simulink model "EV_Pwr_Manager"  (R2013b)
settings: Solver=FixedStepDiscrete  StartTime=0.0  StopTime=inf  RelTol=1e-3
InitFcn:
  | %EV_Param_Update
  | % update the number of strings (discretized)
  | numStrings = round(Opti_numStrings);
  | %disp(['Number of strings: ' num2str(numStrings)])
  | % update the effective capacity based on the number of strings
  | EV_Param.Battery_Det.Rated_Capacity = 28.5*numStrings; %A*hr
  | EV_Param.Battery_Det.DP = 1.5*fliplr([1500 1500 1600 1450 1325 1125 925 675 425 175 ])./8*EV_Param.Battery_Det.Rated_Capacity; % 8 comes from the 8Ahr rated batter data used (normalize and rescale to the rated capacity
  | EV_Param.Battery_Det.CP = fliplr([25 100 200 250 375 550 750 950 1125 1150])./8*EV_Param.Battery_Det.Rated_Capacity;
  | 
  | % update the number of cells in a string (discretized)
  | numSeriesCells = round(Opti_numSeriesCells);
  | %disp(['Number of cells in a string: ' num2str(numSeriesCells)])
  | % update the nominal string volage and charge deficit
  | EV_Param.Battery_Det.Nominal_Voltage = numSeriesCells*cellVolts;
  | BatteryParams(1).Qe_init = 0;%EV_Param.Battery_Det.Rated_Capacity*(1-EV_Param.Battery_Det.Initial_SOC/100); %Ampere*hours
  | 
  | % update the total number of cells, battery pack mass and total vehicle
  | % mass
  | total_cells = numSeriesCells*numStrings;
  | %disp(['Total Number of cells: ' num2str(total_cells)])
  | EV_Param.BatteryMass = BatteryParams(1).cell_mass*total_cells;
  | %disp(['Total Battery Pack Mass: ' num2str(EV_Param.BatteryMass)])
  | EV_Param.Vehicle.Mass = 1300+EV_Param.BatteryMass;
  | 
  | % update the driveline gear ratio
  | EV_Param.Vehicle.Engine_Vehicle_Gear_Ratio = Opti_Vehicle_Gear_Ratio;
  | %disp(['Driveline gear ratio: ' num2str(Opti_Vehicle_Gear_Ratio)])
  | %disp('EV_Pwr_Manager has been initialized')
values from neighbouring files (symbols this model uses):
  ctrlConst = struct    [applicationData.m]
undefined symbols (not defined in the file or in its folder): brake_cmd_table, decel_cmd_vec, DiscIntNeverNeededParam, Motor_Limits, Motor_Spd_Ref_radps, regen_pwr_vec
libraries: simulink x13
settings Model: PauseTimes=13.1  Creator=rchladny  LastModifiedBy=rchladny
settings DataIOCC: SaveOutput=off  SaveTime=off
settings OptimizationCC: InlineParams=on  UseSpecifiedMinMax=on  ZeroExternalMemoryAtStartup=off  NoFixptDivByZeroProtection=on  EfficientFloat2IntCast=on  OptimizeModelRefInitCode=on  LifeSpan=Inf
settings DebuggingCC: InheritedTsInSrcMsg=none  ParameterPrecisionLossMsg=none  UnknownTsInhSupMsg=none
settings HardwareCC: ProdBitPerChar=16  ProdBitPerInt=16  ProdBitPerPointer=16  ProdLargestAtomicInteger=Integer  ProdIntDivRoundTo=Zero  ProdEndianess=LittleEndian  ProdWordSize=16  ProdHWDeviceType=Texas Instruments->C2000  TargetLongLongMode=on  TargetIntDivRoundTo=Zero  TargetEndianess=LittleEndian  TargetHWDeviceType=Generic->MATLAB Host Computer  ProdEqTarget=off
settings ModelReferenceCC: ModelReferenceNumInstancesAllowed=Single
settings RTWCC: SystemTargetFile=ert.tlc  TemplateMakefile=ert_default_tmf  Description=Embedded Coder  ProcessScript=ert_make_rtw_hook
settings CodeAppCC: IgnoreCustomStorageClasses=off
settings ERTTargetCC: CodeReplacementLibrary=ANSI_C  GenerateSampleERTMain=on  ERTCustomFileTemplate=example_file_process.tlc

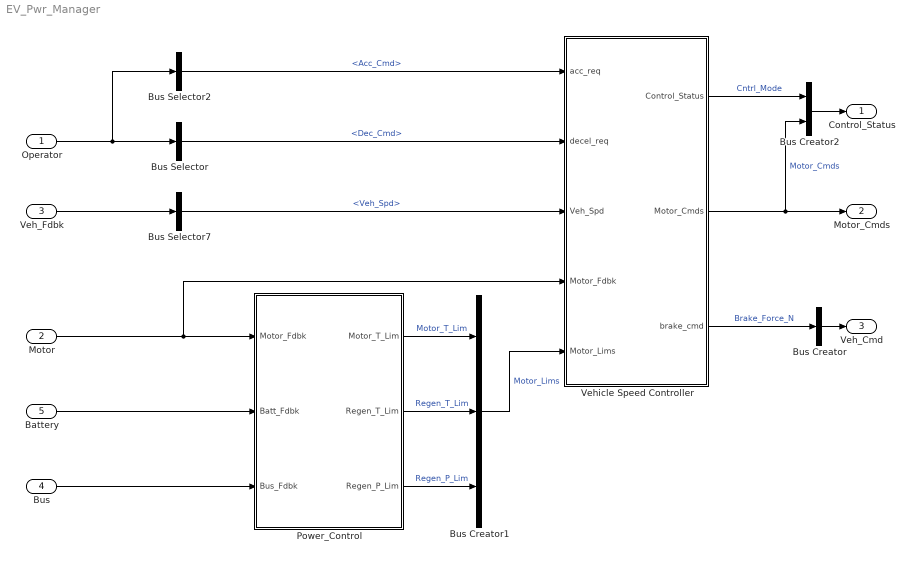
== system EV_Pwr_Manager ==
  Operator : Inport  OutDataTypeStr=Bus: Op_Cmds
  Motor : Inport  Port=2  OutDataTypeStr=Bus: Motor_Sys_Fdbk  BusOutputAsStruct=on
  Veh_Fdbk : Inport  Port=3  OutDataTypeStr=Bus: Veh_Fdbk
  Bus : Inport  Port=4  OutDataTypeStr=Bus: Bus_Fdbk  BusOutputAsStruct=on
  Battery : Inport  Port=5  OutDataTypeStr=Bus: Batt_Fdbk  BusOutputAsStruct=on
  Bus Creator : BusCreator  Inputs=1
  Bus Creator1 : BusCreator  Inputs=3
  Bus Creator2 : BusCreator  Inputs=2
  Bus Selector : BusSelector  OutputSignals=Dec_Cmd
  Bus Selector2 : BusSelector  OutputSignals=Acc_Cmd
  Bus Selector7 : BusSelector  OutputSignals=Veh_Spd
  Power_Control : Subsystem
  Vehicle Speed Controller : Subsystem
  Control_Status : Outport  OutDataTypeStr=Bus: Cntrl_Status
  Motor_Cmds : Outport  Port=2  OutDataTypeStr=Bus: Motor_Cmds
  Veh_Cmd : Outport  Port=3  OutDataTypeStr=Bus: Veh_Cmds
  wires:
  Vehicle Speed Controller/2(Motor_Cmds) -> Bus Creator2/2, Motor_Cmds/1  "Motor_Cmds"
  Power_Control/1(Motor_T_Lim) -> Bus Creator1/1  "Motor_T_Lim"
  Power_Control/2(Regen_T_Lim) -> Bus Creator1/2  "Regen_T_Lim"
  Bus Creator1/1 -> Vehicle Speed Controller/5(Motor_Lims)  "Motor_Lims"
  Power_Control/3(Regen_P_Lim) -> Bus Creator1/3  "Regen_P_Lim"
  Motor/1 -> Vehicle Speed Controller/4(Motor_Fdbk), Power_Control/1(Motor_Fdbk)
  Battery/1 -> Power_Control/2(Batt_Fdbk)
  Bus/1 -> Power_Control/3(Bus_Fdbk)
  Vehicle Speed Controller/1(Control_Status) -> Bus Creator2/1  "Cntrl_Mode"
  Veh_Fdbk/1 -> Bus Selector7/1
  Bus Creator2/1 -> Control_Status/1
  Bus Selector/1 -> Vehicle Speed Controller/2(decel_req)  "<Dec_Cmd>"
  Bus Selector2/1 -> Vehicle Speed Controller/1(acc_req)  "<Acc_Cmd>"
  Operator/1 -> Bus Selector2/1, Bus Selector/1
  Vehicle Speed Controller/3(brake_cmd) -> Bus Creator/1  "Brake_Force_N"
  Bus Creator/1 -> Veh_Cmd/1
  Bus Selector7/1 -> Vehicle Speed Controller/3(Veh_Spd)  "<Veh_Spd>"

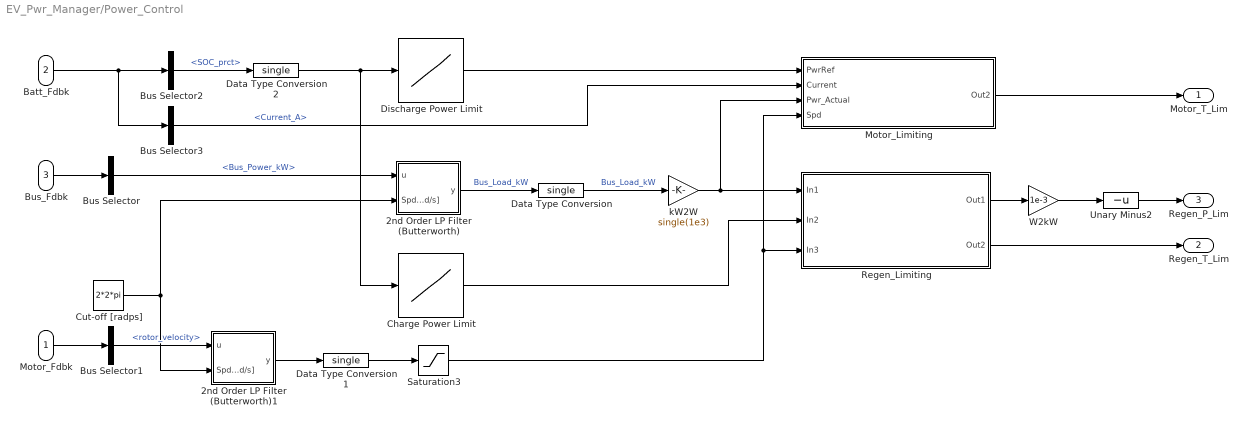
== system EV_Pwr_Manager/Power_Control ==
  Motor_Fdbk : Inport  OutDataTypeStr=Bus: Motor_Sys_Fdbk
  Batt_Fdbk : Inport  Port=2  OutDataTypeStr=Bus: Batt_Fdbk
  Bus_Fdbk : Inport  Port=3  OutDataTypeStr=Bus: Bus_Fdbk
  2nd Order LP Filter (Butterworth) : Subsystem  mask{DT=EV_Param.Control.Pwr_Cntrl_TS}
      mask prompts: DT "Sampe Time"
      mask Display:
      | plot([0 0],[0 1]);
      | plot([0 1],[0 0]);
      | plot([0 .5 .75 1],[1 1 .7071 .01]);
  2nd Order LP Filter (Butterworth)1 : Subsystem  mask{DT=EV_Param.Control.Pwr_Cntrl_TS}
      mask prompts: DT "Sampe Time"
      mask Display:
      | plot([0 0],[0 1]);
      | plot([0 1],[0 0]);
      | plot([0 .5 .75 1],[1 1 .7071 .01]);
  Bus Selector : BusSelector  OutputSignals=Bus_Power_kW
  Bus Selector1 : BusSelector  OutputSignals=Motor_Fdbk.rotor_velocity
  Bus Selector2 : BusSelector  OutputSignals=SOC_prct
  Bus Selector3 : BusSelector  OutputSignals=Current_A
  Charge Power Limit : Lookup_n-D  NumberOfTableDimensions=1  BreakpointsForDimension1=EV_Param.Battery_Det.SOC  BeginIndexSearchUsingPreviousIndexResult=on  Table=EV_Param.Battery_Det.CP  InternalRulePriority=Speed  RndMeth=Simplest  InputSameDT=on
  Cut-off [radps] : Constant  Value=2*2*pi  OutDataTypeStr=single  SampleTime=-1
  Data Type Conversion : DataTypeConversion  OutDataTypeStr=single
  Data Type Conversion1 : DataTypeConversion  OutDataTypeStr=single
  Data Type Conversion2 : DataTypeConversion  OutDataTypeStr=single
  Discharge Power Limit : Lookup_n-D  NumberOfTableDimensions=1  BreakpointsForDimension1=EV_Param.Battery_Det.SOC  BeginIndexSearchUsingPreviousIndexResult=on  Table=EV_Param.Battery_Det.DP  ExtrapMethod=Clip  UseLastTableValue=on  InternalRulePriority=Speed  RndMeth=Simplest  InputSameDT=on
  Motor_Limiting : Subsystem
  Regen_Limiting : Subsystem
  Saturation3 : Saturate  UpperLimit=inf  LowerLimit=100*pi/30
  Unary Minus2 : UnaryMinus
  W2kW : Gain  Gain=1e-3
  kW2W : Gain  Gain=single(1e3)
  Motor_T_Lim : Outport
  Regen_T_Lim : Outport  Port=2
  Regen_P_Lim : Outport  Port=3
  wires:
  Batt_Fdbk/1 -> Bus Selector3/1, Bus Selector2/1
  Cut-off [radps]/1 -> 2nd Order LP Filter (Butterworth)1/2(Spd_Err_Filt_BW [rad/s]), 2nd Order LP Filter (Butterworth)/2(Spd_Err_Filt_BW [rad/s])
  kW2W/1 -> Motor_Limiting/3(Pwr_Actual), Regen_Limiting/1(In1)
  W2kW/1 -> Unary Minus2/1
  Unary Minus2/1 -> Regen_P_Lim/1
  Saturation3/1 -> Motor_Limiting/4(Spd), Regen_Limiting/3(In3)
  Bus_Fdbk/1 -> Bus Selector/1
  2nd Order LP Filter (Butterworth)/1(y) -> Data Type Conversion/1  "Bus_Load_kW"
  Data Type Conversion/1 -> kW2W/1  "Bus_Load_kW"
  Bus Selector/1 -> 2nd Order LP Filter (Butterworth)/1(u)  "<Bus_Power_kW>"
  Motor_Fdbk/1 -> Bus Selector1/1
  Bus Selector1/1 -> 2nd Order LP Filter (Butterworth)1/1(u)  "<rotor_velocity>"
  Bus Selector2/1 -> Data Type Conversion2/1  "<SOC_prct>"
  2nd Order LP Filter (Butterworth)1/1(y) -> Data Type Conversion1/1
  Data Type Conversion1/1 -> Saturation3/1
  Data Type Conversion2/1 -> Charge Power Limit/1, Discharge Power Limit/1
  Discharge Power Limit/1 -> Motor_Limiting/1(PwrRef)
  Bus Selector3/1 -> Motor_Limiting/2(Current)  "<Current_A>"
  Motor_Limiting/1(Out2) -> Motor_T_Lim/1
  Charge Power Limit/1 -> Regen_Limiting/2(In2)
  Regen_Limiting/1(Out1) -> W2kW/1
  Regen_Limiting/2(Out2) -> Regen_T_Lim/1

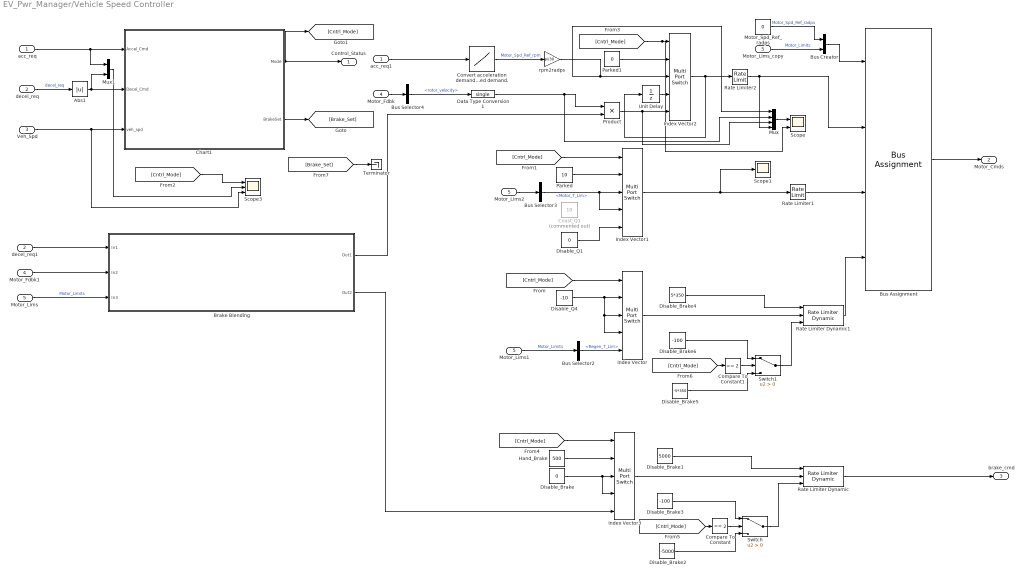
== system EV_Pwr_Manager/Vehicle Speed Controller ==
  acc_req : Inport
  decel_req : Inport  Port=2
  Veh_Spd : Inport  Port=3  OutDataTypeStr=single
  Motor_Fdbk : Inport  Port=4
  Motor_Lims : Inport  Port=5
  Abs1 : Abs
  Brake Blending : Subsystem
  Bus Assignment : BusAssignment  AssignedSignals=Motor_Spd_Ref_radps,Motor_Limits.Motor_T_Lim,Motor_Limits.Regen_T_Lim
  Bus Creator : BusCreator  Inputs=2
  Bus Selector2 : BusSelector  OutputSignals=Regen_T_Lim
  Bus Selector3 : BusSelector  OutputSignals=Motor_T_Lim
  Bus Selector4 : BusSelector  OutputSignals=Motor_Fdbk.rotor_velocity
  Chart1 : Stateflow chart  TreatAsAtomicUnit=on
  Coast_Q1 : Constant  Commented=on  Value=10  OutDataTypeStr=single
  Compare To Constant : simulink/Logic and Bit Operations/Compare To Constant  relop===  const=2  OutDataTypeStr=boolean
  Compare To Constant1 : simulink/Logic and Bit Operations/Compare To Constant  relop===  const=2  OutDataTypeStr=boolean
  Convert acceleration demand to motor speed demand. : Lookup_n-D  NumberOfTableDimensions=1  BreakpointsForDimension1=[0 1]  BeginIndexSearchUsingPreviousIndexResult=on  Table=[0 2500]*.8  InputSameDT=on
  Data Type Conversion1 : DataTypeConversion  OutDataTypeStr=single
  Disable_Brake : Constant  Value=0  OutDataTypeStr=single
  Disable_Brake1 : Constant  Value=5000  OutDataTypeStr=single  SampleTime=-1
  Disable_Brake2 : Constant  Value=-5000  OutDataTypeStr=single  SampleTime=-1
  Disable_Brake3 : Constant  Value=-100  OutDataTypeStr=single  SampleTime=-1
  Disable_Brake4 : Constant  Value=5*350  OutDataTypeStr=single  SampleTime=-1
  Disable_Brake5 : Constant  Value=-5*350  OutDataTypeStr=single  SampleTime=-1
  Disable_Brake6 : Constant  Value=-100  OutDataTypeStr=single  SampleTime=-1
  Disable_Q1 : Constant  Value=0  OutDataTypeStr=single
  Disable_Q4 : Constant  Value=-10  OutDataTypeStr=single
  Hand_Brake : Constant  Value=500  OutDataTypeStr=single
  Index Vector{,1..3} (4 alike) : MultiPortSwitch  DataPortOrder=Zero-based contiguous  Inputs=4  zeroidx=on
  Motor_Fdbk1 : InportShadow  Port=4
  Motor_Lims1 : InportShadow  Port=5
  Motor_Lims2 : InportShadow  Port=5
  Motor_Lims_copy : InportShadow  Port=5
  Motor_Spd_Ref_radps : Constant  Value=0  OutDataTypeStr=single
  Mux : Mux
  Mux1 : Mux  Inputs=2
  Parked : Constant  Value=10  OutDataTypeStr=single
  Parked1 : Constant  Value=0  OutDataTypeStr=single
  Product : Product
  Rate Limiter Dynamic : simulink/Discontinuities/Rate Limiter Dynamic
  Rate Limiter Dynamic1 : simulink/Discontinuities/Rate Limiter Dynamic
  Rate Limiter1 : RateLimiter  RisingSlewLimit=350*5  FallingSlewLimit=-350*5  SampleTimeMode=inherited
  Rate Limiter2 : RateLimiter  RisingSlewLimit=2000  FallingSlewLimit=-70  SampleTimeMode=inherited
  Scope : Scope  NumInputPorts=2
      settings: YMin=-50~-5  YMax=900~5
  Scope1 : Scope
  Scope3 : Scope  NumInputPorts=3
      settings: YMin=0~0~0  YMax=1~1~275  SaveName=ScopeData23
  Switch : Switch  Criteria=u2 > Threshold
  Switch1 : Switch  Criteria=u2 > Threshold
  Terminator : Terminator
  Unit Delay : UnitDelay  SampleTime=-1
  acc_req1 : InportShadow
  decel_req1 : InportShadow  Port=2
  rpm2radps : Gain  Gain=pi/30
  Control_Status : Outport  InitialOutput=0
  Motor_Cmds : Outport  Port=2  OutDataTypeStr=Bus: Motor_Cmds
  brake_cmd : Outport  Port=3  InitialOutput=0
  wires:
  rpm2radps/1 -> Index Vector2/3, Mux/1
  decel_req/1 -> Abs1/1  "decel_req"
  Convert acceleration demand to motor speed demand./1 -> rpm2radps/1  "Motor_Spd_Ref_rpm"
  Chart1/1(Mode) -> [Cntrl_Mode], Control_Status/1
  Chart1/2(BrakeSet) -> [Brake_Set]
  acc_req/1 -> Mux1/1, Chart1/1(Accel_Cmd)
  Abs1/1 -> Mux1/2, Chart1/2(Decel_Cmd)
  Veh_Spd/1 -> Scope3/3, Chart1/3(veh_spd)
  Motor_Lims_copy/1 -> Bus Creator/2  "Motor_Limits"
  Bus Assignment/1 -> Motor_Cmds/1
  Motor_Spd_Ref_radps/1 -> Bus Creator/1  "Motor_Spd_Ref_radps"
  Bus Creator/1 -> Bus Assignment/1
  Index Vector/1 -> Rate Limiter Dynamic1/2
  Disable_Q4/1 -> Index Vector/4, Index Vector/3, Index Vector/2
  [Cntrl_Mode] -> Index Vector/1
  Rate Limiter Dynamic1/1 -> Bus Assignment/4
  [Cntrl_Mode] -> Index Vector1/1
  Index Vector1/1 -> Scope1/1, Rate Limiter1/1
  Rate Limiter1/1 -> Bus Assignment/3
  Parked/1 -> Index Vector1/2
  [Cntrl_Mode] -> Scope/2, Index Vector2/1
  Parked1/1 -> Index Vector2/2
  Index Vector2/1 -> Unit Delay/1, Rate Limiter2/1
  Bus Selector4/1 -> Data Type Conversion1/1  "<rotor_velocity>"
  Motor_Lims1/1 -> Bus Selector2/1  "Motor_Limits"
  Bus Selector2/1 -> Index Vector/5  "<Regen_T_Lim>"
  Motor_Lims2/1 -> Bus Selector3/1
  Bus Selector3/1 -> Index Vector1/4, Index Vector1/3  "<Motor_T_Lim>"
  Product/1 -> Mux/3, Index Vector2/5
  Mux1/1 -> Scope3/2
  Index Vector3/1 -> Rate Limiter Dynamic/2
  Disable_Brake/1 -> Index Vector3/3, Index Vector3/4
  [Cntrl_Mode] -> Index Vector3/1
  Hand_Brake/1 -> Index Vector3/2
  Rate Limiter2/1 -> Mux/4, Bus Assignment/2
  [Cntrl_Mode] -> Scope3/1
  Motor_Fdbk/1 -> Bus Selector4/1
  Data Type Conversion1/1 -> Product/1, Mux/2
  Rate Limiter Dynamic/1 -> brake_cmd/1
  Switch/1 -> Rate Limiter Dynamic/3
  Compare To Constant/1 -> Switch/2
  [Cntrl_Mode] -> Compare To Constant/1
  Disable_Brake1/1 -> Rate Limiter Dynamic/1
  Disable_Brake2/1 -> Switch/3
  Disable_Brake3/1 -> Switch/1
  Switch1/1 -> Rate Limiter Dynamic1/3
  Compare To Constant1/1 -> Switch1/2
  [Cntrl_Mode] -> Compare To Constant1/1
  Disable_Brake4/1 -> Rate Limiter Dynamic1/1
  Disable_Brake5/1 -> Switch1/3
  Disable_Brake6/1 -> Switch1/1
  Disable_Q1/1 -> Index Vector1/5
  decel_req1/1 -> Brake Blending/1(In1)
  Motor_Fdbk1/1 -> Brake Blending/2(In2)
  Motor_Lims/1 -> Brake Blending/3(In3)  "Motor_Limits"
  Brake Blending/1(Out1) -> Product/2
  Brake Blending/2(Out2) -> Index Vector3/5
  [Brake_Set] -> Terminator/1
  Mux/1 -> Scope/1
  Unit Delay/1 -> Index Vector2/4
  acc_req1/1 -> Convert acceleration demand to motor speed demand./1

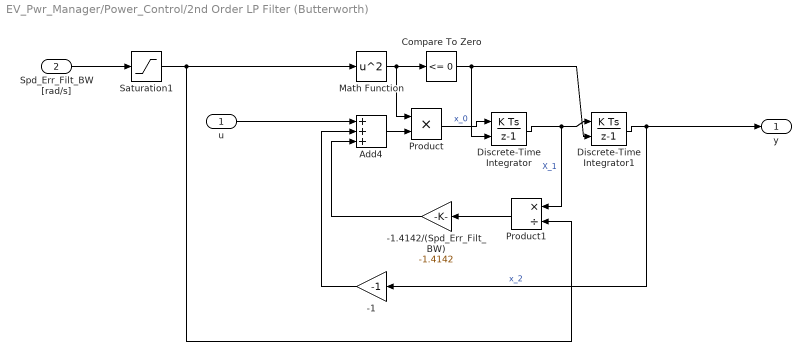
== system EV_Pwr_Manager/Power_Control/2nd Order LP Filter (Butterworth) ==
  u : Inport
  Spd_Err_Filt_BW [rad/s] : Inport  Port=2
  -1 : Gain  Gain=-1
  -1.4142/(Spd_Err_Filt_BW) : Gain  Gain=-1.4142
  Add4 : Sum  Inputs=+++
  Compare To Zero : simulink/Logic and Bit Operations/Compare To Zero  relop=<=  OutDataTypeStr=uint8
  Discrete-Time Integrator : DiscreteIntegrator  ExternalReset=rising  SampleTime=DT  ICPrevOutput=DiscIntNeverNeededParam  ICPrevScaledInput=DiscIntNeverNeededParam
  Discrete-Time Integrator1 : DiscreteIntegrator  ExternalReset=rising  SampleTime=DT  ICPrevOutput=DiscIntNeverNeededParam  ICPrevScaledInput=DiscIntNeverNeededParam
  Math Function : Math  Operator=square  SaturateOnIntegerOverflow=on
  Product : Product  RndMeth=Zero
  Product1 : Product  Inputs=*/  RndMeth=Zero
  Saturation1 : Saturate  UpperLimit=2*pi*5000  LowerLimit=.001
  y : Outport
  wires:
  Add4/1 -> Product/2
  Discrete-Time Integrator/1 -> Product1/1, Discrete-Time Integrator1/1  "X_1"
  Discrete-Time Integrator1/1 -> -1/1, y/1  "x_2"
  -1.4142/(Spd_Err_Filt_BW)/1 -> Add4/3
  -1/1 -> Add4/2
  Product/1 -> Discrete-Time Integrator/1  "x_0"
  u/1 -> Add4/1
  Math Function/1 -> Product/1, Compare To Zero/1
  Spd_Err_Filt_BW [rad/s]/1 -> Saturation1/1
  Product1/1 -> -1.4142/(Spd_Err_Filt_BW)/1
  Compare To Zero/1 -> Discrete-Time Integrator/2, Discrete-Time Integrator1/2
  Saturation1/1 -> Math Function/1, Product1/2

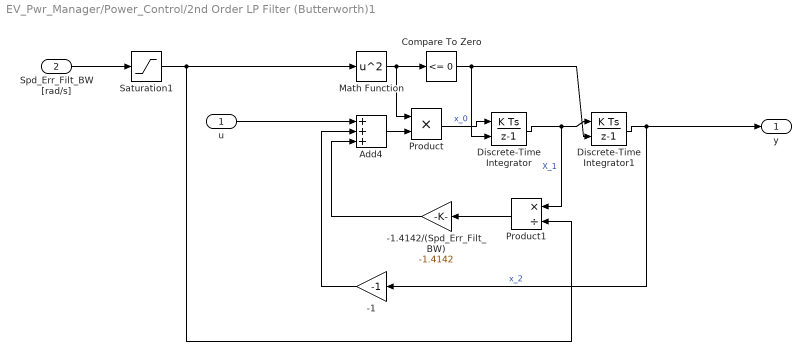
== system EV_Pwr_Manager/Power_Control/2nd Order LP Filter (Butterworth)1 ==
  u : Inport
  Spd_Err_Filt_BW [rad/s] : Inport  Port=2
  -1 : Gain  Gain=-1
  -1.4142/(Spd_Err_Filt_BW) : Gain  Gain=-1.4142
  Add4 : Sum  Inputs=+++
  Compare To Zero : simulink/Logic and Bit Operations/Compare To Zero  relop=<=  OutDataTypeStr=uint8
  Discrete-Time Integrator : DiscreteIntegrator  ExternalReset=rising  SampleTime=DT  ICPrevOutput=DiscIntNeverNeededParam  ICPrevScaledInput=DiscIntNeverNeededParam
  Discrete-Time Integrator1 : DiscreteIntegrator  ExternalReset=rising  SampleTime=DT  ICPrevOutput=DiscIntNeverNeededParam  ICPrevScaledInput=DiscIntNeverNeededParam
  Math Function : Math  Operator=square  SaturateOnIntegerOverflow=on
  Product : Product  RndMeth=Zero
  Product1 : Product  Inputs=*/  RndMeth=Zero
  Saturation1 : Saturate  UpperLimit=2*pi*5000  LowerLimit=.001
  y : Outport
  wires:
  Saturation1/1 -> Product1/2, Math Function/1
  Compare To Zero/1 -> Discrete-Time Integrator1/2, Discrete-Time Integrator/2
  Product1/1 -> -1.4142/(Spd_Err_Filt_BW)/1
  Spd_Err_Filt_BW [rad/s]/1 -> Saturation1/1
  Math Function/1 -> Compare To Zero/1, Product/1
  u/1 -> Add4/1
  Product/1 -> Discrete-Time Integrator/1  "x_0"
  -1/1 -> Add4/2
  -1.4142/(Spd_Err_Filt_BW)/1 -> Add4/3
  Discrete-Time Integrator1/1 -> y/1, -1/1  "x_2"
  Discrete-Time Integrator/1 -> Discrete-Time Integrator1/1, Product1/1  "X_1"
  Add4/1 -> Product/2

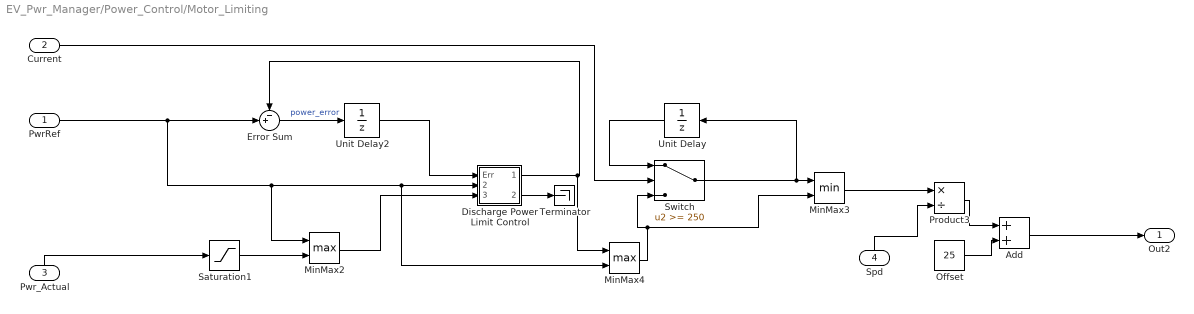
== system EV_Pwr_Manager/Power_Control/Motor_Limiting ==
  PwrRef : Inport
  Current : Inport  Port=2
  Pwr_Actual : Inport  Port=3
  Spd : Inport  Port=4
  Add : Sum
  Discharge Power Limit Control : Subsystem
      mask Display:
      | disp('PI(z)')
      | port_label('input',1, '');
      | port_label('output',1, '');
  Error Sum : Sum  Inputs=-+|  OutMin=-2*ctrlConst.VelocityMax  OutMax=2*ctrlConst.VelocityMax  OutDataTypeStr=DT_PRECISION_LO
  MinMax2 : MinMax  Function=max  Inputs=2
  MinMax3 : MinMax  Inputs=2
  MinMax4 : MinMax  Function=max  Inputs=2
  Offset : Constant  Value=25  OutDataTypeStr=single  SampleTime=-1
  Product3 : Product  Inputs=*/
  Saturation1 : Saturate  UpperLimit=100e3  LowerLimit=0
  Switch : Switch  Threshold=250
  Terminator : Terminator
  Unit Delay : UnitDelay  SampleTime=-1
  Unit Delay2 : UnitDelay  SampleTime=-1
  Out2 : Outport
  wires:
  Pwr_Actual/1 -> Saturation1/1
  Spd/1 -> Product3/2
  Error Sum/1 -> Unit Delay2/1  "power_error"
  Unit Delay2/1 -> Discharge Power Limit Control/1(Err)
  Product3/1 -> Add/1
  Saturation1/1 -> MinMax2/2
  Add/1 -> Out2/1
  Offset/1 -> Add/2
  Discharge Power Limit Control/1(Out) -> MinMax4/1, Error Sum/1
  PwrRef/1 -> Error Sum/2, MinMax2/1, MinMax4/2, Discharge Power Limit Control/2(Power_Min)
  Current/1 -> Switch/2
  Unit Delay/1 -> Switch/1
  MinMax2/1 -> Discharge Power Limit Control/3(Input_Disturbance)
  MinMax4/1 -> MinMax3/2, Switch/3
  Switch/1 -> MinMax3/1, Unit Delay/1
  MinMax3/1 -> Product3/1
  Discharge Power Limit Control/2(Lim_Out) -> Terminator/1

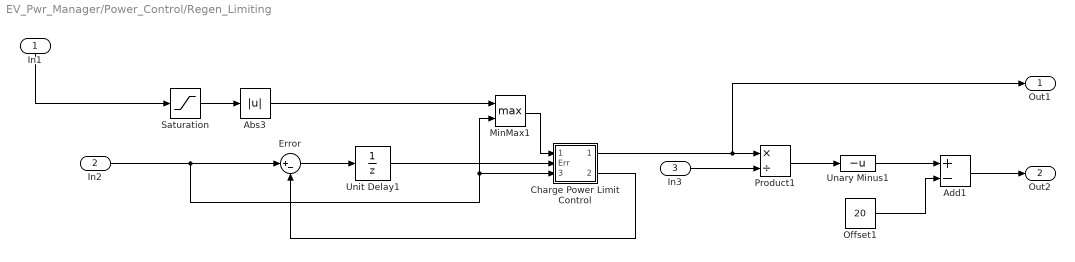
== system EV_Pwr_Manager/Power_Control/Regen_Limiting ==
  In1 : Inport
  In2 : Inport  Port=2
  In3 : Inport  Port=3
  Abs3 : Abs
  Add1 : Sum  Inputs=+-
  Charge Power Limit Control : Subsystem
      mask Display:
      | disp('PI(z)')
      | port_label('input',1, '');
      | port_label('output',1, '');
  Error : Sum  Inputs=|+-  OutMin=-2*ctrlConst.VelocityMax  OutMax=2*ctrlConst.VelocityMax  OutDataTypeStr=DT_PRECISION_LO
  MinMax1 : MinMax  Function=max  Inputs=2
  Offset1 : Constant  Value=20  OutDataTypeStr=single  SampleTime=-1
  Product1 : Product  Inputs=*/
  Saturation : Saturate  UpperLimit=0  LowerLimit=-100e3
  Unary Minus1 : UnaryMinus
  Unit Delay1 : UnitDelay  SampleTime=-1
  Out1 : Outport
  Out2 : Outport  Port=2
  wires:
  In1/1 -> Saturation/1
  In3/1 -> Product1/2
  Error/1 -> Unit Delay1/1
  Charge Power Limit Control/2(Out) -> Error/2
  Unit Delay1/1 -> Charge Power Limit Control/2(Err)
  Saturation/1 -> Abs3/1
  Product1/1 -> Unary Minus1/1
  Unary Minus1/1 -> Add1/1
  Abs3/1 -> MinMax1/1
  Add1/1 -> Out2/1
  In2/1 -> MinMax1/2, Charge Power Limit Control/3(Power_Min), Error/1
  Charge Power Limit Control/1(Lim_Out) -> Out1/1, Product1/1
  MinMax1/1 -> Charge Power Limit Control/1(Input_Disturbance)
  Offset1/1 -> Add1/2

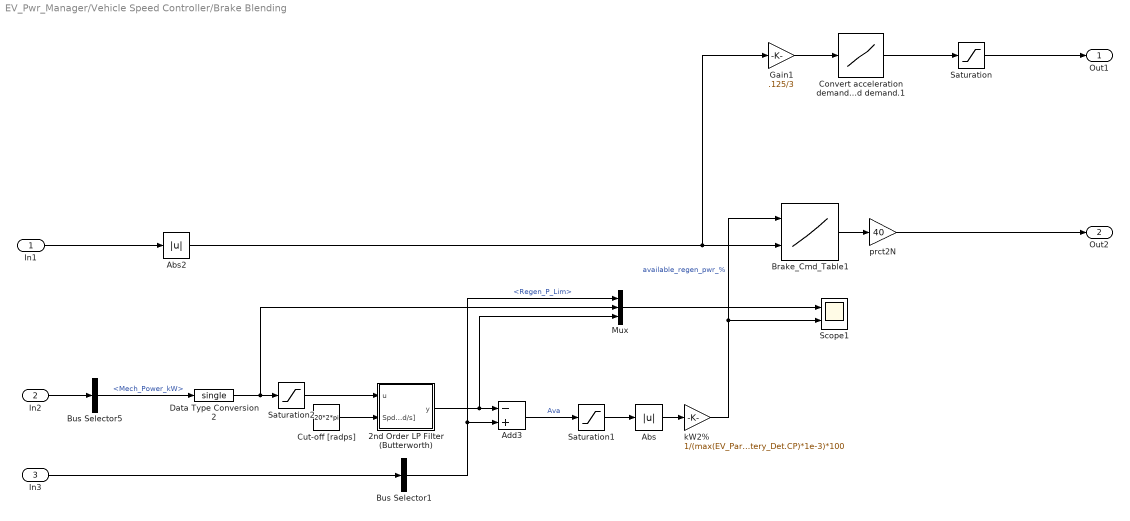
== system EV_Pwr_Manager/Vehicle Speed Controller/Brake Blending ==
  In1 : Inport
  In2 : Inport  Port=2
  In3 : Inport  Port=3
  2nd Order LP Filter (Butterworth) : Subsystem  mask{DT=EV_Param.Control.Pwr_Cntrl_TS}
      mask prompts: DT "Sampe Time"
      mask Display:
      | plot([0 0],[0 1]);
      | plot([0 1],[0 0]);
      | plot([0 .5 .75 1],[1 1 .7071 .01]);
  Abs : Abs
  Abs2 : Abs
  Add3 : Sum  Inputs=-+
  Brake_Cmd_Table1 : Lookup_n-D  BreakpointsForDimension1=regen_pwr_vec  BreakpointsForDimension2=decel_cmd_vec  Table=brake_cmd_table  ExtrapMethod=Clip  UseLastTableValue=on  InternalRulePriority=Speed  RndMeth=Simplest  InputSameDT=on
  Bus Selector1 : BusSelector  OutputSignals=Regen_P_Lim
  Bus Selector5 : BusSelector  OutputSignals=Motor_Fdbk.Mech_Power_kW
  Convert acceleration demand to motor speed demand.1 : Lookup_n-D  NumberOfTableDimensions=1  BreakpointsForDimension1=[0 20]  BeginIndexSearchUsingPreviousIndexResult=on  Table=[1 0]  ExtrapMethod=Clip  UseLastTableValue=on  InputSameDT=on
  Cut-off [radps] : Constant  Value=20*2*pi  OutDataTypeStr=single  SampleTime=-1
  Data Type Conversion2 : DataTypeConversion  OutDataTypeStr=single
  Gain1 : Gain  Gain=.125/3
  Mux : Mux  Inputs=3
  Saturation : Saturate  UpperLimit=1  LowerLimit=0
  Saturation1 : Saturate  UpperLimit=0  LowerLimit=-300
  Saturation2 : Saturate  UpperLimit=0  LowerLimit=-300
  Scope1 : Scope  NumInputPorts=2
      settings: YMin=-12.5~0  YMax=35~105  SaveName=ScopeData24
  kW2% : Gain  Gain=1/(max(EV_Param.Battery_Det.CP)*1e-3)*100
  prct2N : Gain  Gain=40
  Out1 : Outport
  Out2 : Outport  Port=2
  wires:
  In3/1 -> Bus Selector1/1
  Bus Selector1/1 -> Mux/1, Add3/2  "<Regen_P_Lim>"
  Add3/1 -> Saturation1/1  "Ava"
  Cut-off [radps]/1 -> 2nd Order LP Filter (Butterworth)/2(Spd_Err_Filt_BW [rad/s])
  2nd Order LP Filter (Butterworth)/1(y) -> Mux/3, Add3/1
  Saturation1/1 -> Abs/1
  Abs/1 -> kW2%/1
  Saturation2/1 -> 2nd Order LP Filter (Butterworth)/1(u)
  Mux/1 -> Scope1/1
  prct2N/1 -> Out2/1
  Brake_Cmd_Table1/1 -> prct2N/1
  Abs2/1 -> Gain1/1, Brake_Cmd_Table1/2
  In1/1 -> Abs2/1
  kW2%/1 -> Scope1/2, Brake_Cmd_Table1/1  "available_regen_pwr_%"
  Saturation/1 -> Out1/1
  Gain1/1 -> Convert acceleration demand to motor speed demand.1/1
  Convert acceleration demand to motor speed demand.1/1 -> Saturation/1
  Bus Selector5/1 -> Data Type Conversion2/1  "<Mech_Power_kW>"
  In2/1 -> Bus Selector5/1
  Data Type Conversion2/1 -> Mux/2, Saturation2/1

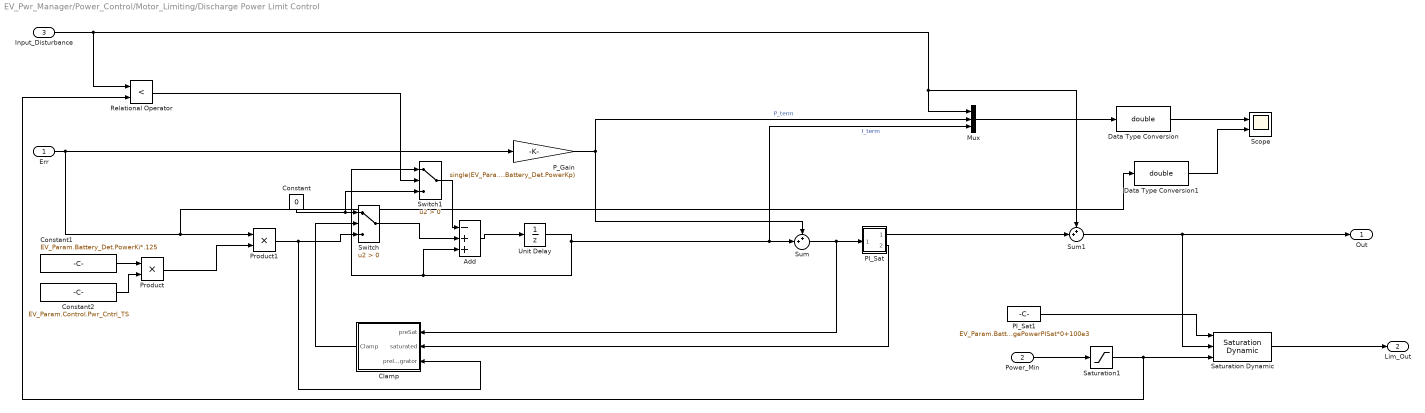
== system EV_Pwr_Manager/Power_Control/Motor_Limiting/Discharge Power Limit Control ==
  Err : Inport
  Power_Min : Inport  Port=2
  Input_Disturbance : Inport  Port=3
  Add : Sum  Inputs=-++  OutMin=-ctrlConst.CurrentMax*2  OutMax=ctrlConst.CurrentMax*2  OutDataTypeStr=DT_PRECISION_HI  SaturateOnIntegerOverflow=on
      settings: AttributesFormatString=-----------------------------\nMin = %<OutMin>\nMax = %<OutMax>\nSat = %<SaturateOnIntegerOverflow>
  Clamp : Subsystem
  Constant : Constant  Value=0  OutDataTypeStr=Inherit: Inherit via back propagation  SampleTime=-1  PreserveConstantTs=on
  Constant1 : Constant  Value=EV_Param.Battery_Det.PowerKi*.125  SampleTime=-1
  Constant2 : Constant  Value=EV_Param.Control.Pwr_Cntrl_TS  OutDataTypeStr=DT_PRECISION_LO  SampleTime=-1
  Data Type Conversion : DataTypeConversion  OutDataTypeStr=double
  Data Type Conversion1 : DataTypeConversion  OutDataTypeStr=double
  Mux : Mux  Inputs=3
  PI_Sat : Subsystem
      mask Display: plot([0.15 0.85],[.5 .5],[.5 .5],[0.05 0.95],0.15+0.7*[0 .25 .75 1],0.05+0.9*[.25 .25 .75 .75]);
  PI_Sat1 : Constant  Value=EV_Param.Battery_Det.DischargePowerPISat*0+100e3  SampleTime=-1  PreserveConstantTs=on
  P_Gain : Gain  Gain=single(EV_Param.Battery_Det.PowerKp)  ParamDataTypeStr=Inherit: Inherit from 'Gain'
      settings: AttributesFormatString=-----------------------------\n%<Gain>
  Product : Product  OutDataTypeStr=single
  Product1 : Product  OutDataTypeStr=single
  Relational Operator : RelationalOperator  Operator=<  OutDataTypeStr=boolean
  Saturation Dynamic : simulink/Discontinuities/Saturation Dynamic  OutMin=[]  OutMax=[]  OutDataTypeStr=Inherit: Same as second input  OutDataType=fixdt(1, 16)  OutScaling=2^-10  DoSatur=off
  Saturation1 : Saturate  UpperLimit=max(EV_Param.Battery_Det.DP)  LowerLimit=0
  Scope : Scope  NumInputPorts=2
      settings: TimeRange=18  YMin=-5000~-52500  YMax=65000~0  SaveName=ScopeData19
  Sum : Sum  Inputs=++|
  Sum1 : Sum  Inputs=++|
  Switch : Switch  Criteria=u2 > Threshold  InputSameDT=on
  Switch1 : Switch  Criteria=u2 > Threshold  InputSameDT=on
  Unit Delay : UnitDelay  SampleTime=-1
  Out : Outport
  Lim_Out : Outport  Port=2
  wires:
  Switch/1 -> Add/2
  PI_Sat/2(saturated) -> Clamp/2(saturated)
  Err/1 -> Product1/1, Data Type Conversion1/1, P_Gain/1
  P_Gain/1 -> Mux/2, Sum/1  "P_term"
  Add/1 -> Unit Delay/1
  Unit Delay/1 -> Switch1/1, Add/3, Mux/3, Sum/2  "I_term"
  Constant/1 -> Switch1/3, Switch/1
  Clamp/1(Clamp) -> Switch/2
  Constant1/1 -> Product/1
  Constant2/1 -> Product/2
  Sum1/1 -> Saturation Dynamic/2, Out/1
  Power_Min/1 -> Saturation1/1
  Mux/1 -> Data Type Conversion/1
  PI_Sat1/1 -> Saturation Dynamic/1
  Input_Disturbance/1 -> Relational Operator/1, Mux/1, Sum1/1
  Sum/1 -> PI_Sat/1(In1), Clamp/1(preSat)
  Data Type Conversion/1 -> Scope/1
  PI_Sat/1(Out1) -> Sum1/2
  Product/1 -> Product1/2
  Product1/1 -> Clamp/3(preIntegrator), Switch/3
  Data Type Conversion1/1 -> Scope/2
  Saturation1/1 -> Relational Operator/2, Saturation Dynamic/3
  Saturation Dynamic/1 -> Lim_Out/1
  Switch1/1 -> Add/1
  Relational Operator/1 -> Switch1/2

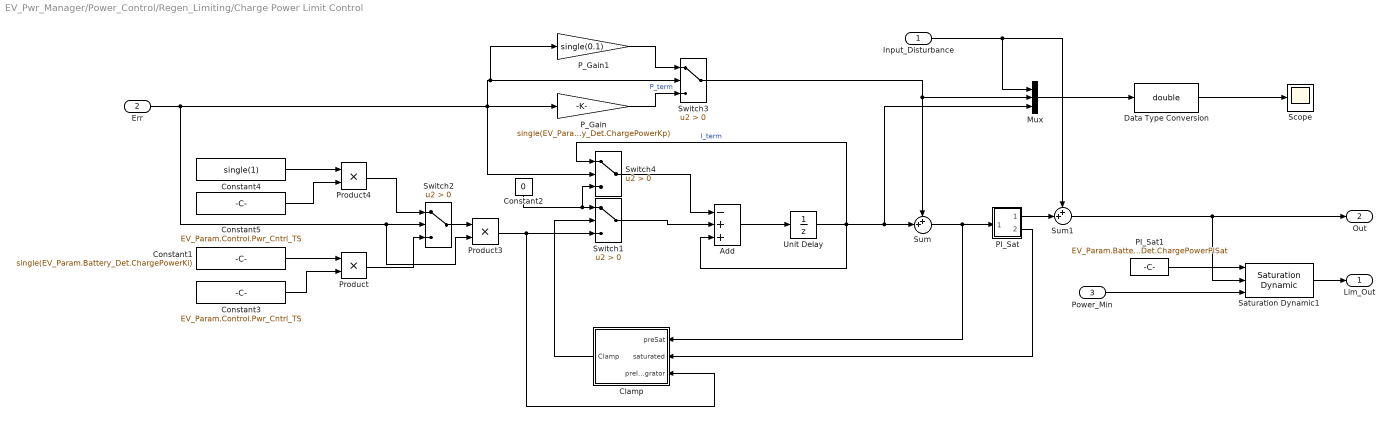
== system EV_Pwr_Manager/Power_Control/Regen_Limiting/Charge Power Limit Control ==
  Input_Disturbance : Inport
  Err : Inport  Port=2
  Power_Min : Inport  Port=3
  Add : Sum  Inputs=-++  OutMin=-ctrlConst.CurrentMax*2  OutMax=ctrlConst.CurrentMax*2  OutDataTypeStr=DT_PRECISION_HI  SaturateOnIntegerOverflow=on
      settings: AttributesFormatString=-----------------------------\nMin = %<OutMin>\nMax = %<OutMax>\nSat = %<SaturateOnIntegerOverflow>
  Clamp : Subsystem
  Constant1 : Constant  Value=single(EV_Param.Battery_Det.ChargePowerKi)  SampleTime=-1
  Constant2 : Constant  Value=0  OutDataTypeStr=Inherit: Inherit via back propagation  PreserveConstantTs=on
  Constant3 : Constant  Value=EV_Param.Control.Pwr_Cntrl_TS  OutDataTypeStr=DT_PRECISION_LO  SampleTime=-1
  Constant4 : Constant  Value=single(1)  SampleTime=-1
  Constant5 : Constant  Value=EV_Param.Control.Pwr_Cntrl_TS  OutDataTypeStr=DT_PRECISION_LO  SampleTime=-1
  Data Type Conversion : DataTypeConversion  OutDataTypeStr=double
  Mux : Mux  Inputs=3
  PI_Sat : Subsystem
      mask Display: plot([0.15 0.85],[.5 .5],[.5 .5],[0.05 0.95],0.15+0.7*[0 .25 .75 1],0.05+0.9*[.25 .25 .75 .75]);
  PI_Sat1 : Constant  Value=EV_Param.Battery_Det.ChargePowerPISat  PreserveConstantTs=on
  P_Gain : Gain  Gain=single(EV_Param.Battery_Det.ChargePowerKp)  ParamDataTypeStr=Inherit: Inherit from 'Gain'
      settings: AttributesFormatString=-----------------------------\n%<Gain>
  P_Gain1 : Gain  Gain=single(0.1)  ParamDataTypeStr=Inherit: Inherit from 'Gain'
      settings: AttributesFormatString=-----------------------------\n%<Gain>
  Product : Product  OutDataTypeStr=single
  Product3 : Product  OutDataTypeStr=single
  Product4 : Product
  Saturation Dynamic1 : simulink/Discontinuities/Saturation Dynamic  OutMin=[]  OutMax=[]  OutDataTypeStr=Inherit: Same as second input  OutDataType=fixdt(1, 16)  OutScaling=2^-10  DoSatur=off
  Scope : Scope
      settings: TimeRange=18  YMin=-75000  YMax=150000
  Sum : Sum  Inputs=++|
  Sum1 : Sum  Inputs=++|
  Switch{1..4} (4 alike) : Switch  Criteria=u2 > Threshold  InputSameDT=on
  Unit Delay : UnitDelay  SampleTime=-1
  Lim_Out : Outport
  Out : Outport  Port=2
  wires:
  Switch1/1 -> Add/2
  PI_Sat/2(saturated) -> Clamp/2(saturated)
  Add/1 -> Unit Delay/1
  Unit Delay/1 -> Add/3, Switch4/1, Mux/3, Sum/2  "I_term"
  Sum1/1 -> Out/1, Saturation Dynamic1/2
  Power_Min/1 -> Saturation Dynamic1/3
  Mux/1 -> Data Type Conversion/1
  PI_Sat1/1 -> Saturation Dynamic1/1
  Input_Disturbance/1 -> Mux/1, Sum1/1
  Sum/1 -> PI_Sat/1(In1), Clamp/1(preSat)
  Saturation Dynamic1/1 -> Lim_Out/1
  Data Type Conversion/1 -> Scope/1
  PI_Sat/1(Out1) -> Sum1/2
  Err/1 -> Product3/2, Switch2/2, Switch4/2, P_Gain1/1, Switch3/2, P_Gain/1
  Constant2/1 -> Switch4/3, Switch1/1
  Clamp/1(Clamp) -> Switch1/2
  Constant1/1 -> Product/1
  Constant3/1 -> Product/2
  Product/1 -> Switch2/3
  Constant4/1 -> Product4/1
  Constant5/1 -> Product4/2
  Product4/1 -> Switch2/1
  Switch2/1 -> Product3/1
  Product3/1 -> Clamp/3(preIntegrator), Switch1/3
  P_Gain/1 -> Switch3/3  "P_term"
  Switch3/1 -> Mux/2, Sum/1
  P_Gain1/1 -> Switch3/1
  Switch4/1 -> Add/1

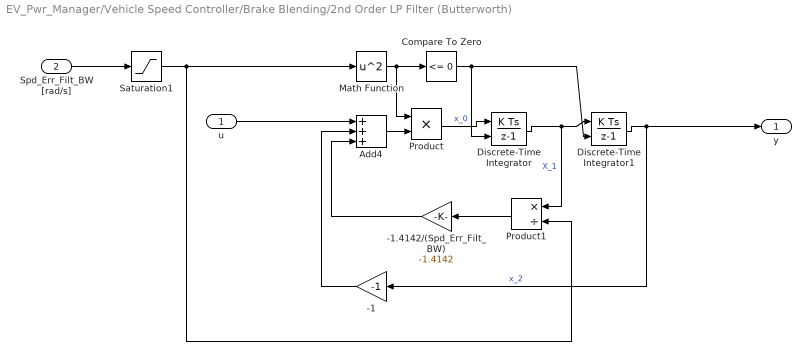
== system EV_Pwr_Manager/Vehicle Speed Controller/Brake Blending/2nd Order LP Filter (Butterworth) ==
  u : Inport
  Spd_Err_Filt_BW [rad/s] : Inport  Port=2
  -1 : Gain  Gain=-1
  -1.4142/(Spd_Err_Filt_BW) : Gain  Gain=-1.4142
  Add4 : Sum  Inputs=+++
  Compare To Zero : simulink/Logic and Bit Operations/Compare To Zero  relop=<=  OutDataTypeStr=uint8
  Discrete-Time Integrator : DiscreteIntegrator  ExternalReset=rising  SampleTime=DT  ICPrevOutput=DiscIntNeverNeededParam  ICPrevScaledInput=DiscIntNeverNeededParam
  Discrete-Time Integrator1 : DiscreteIntegrator  ExternalReset=rising  SampleTime=DT  ICPrevOutput=DiscIntNeverNeededParam  ICPrevScaledInput=DiscIntNeverNeededParam
  Math Function : Math  Operator=square  SaturateOnIntegerOverflow=on
  Product : Product  RndMeth=Zero
  Product1 : Product  Inputs=*/  RndMeth=Zero
  Saturation1 : Saturate  UpperLimit=2*pi*5000  LowerLimit=.001
  y : Outport
  wires:
  Add4/1 -> Product/2
  Discrete-Time Integrator/1 -> Product1/1, Discrete-Time Integrator1/1  "X_1"
  Discrete-Time Integrator1/1 -> -1/1, y/1  "x_2"
  -1.4142/(Spd_Err_Filt_BW)/1 -> Add4/3
  -1/1 -> Add4/2
  Product/1 -> Discrete-Time Integrator/1  "x_0"
  u/1 -> Add4/1
  Math Function/1 -> Product/1, Compare To Zero/1
  Spd_Err_Filt_BW [rad/s]/1 -> Saturation1/1
  Product1/1 -> -1.4142/(Spd_Err_Filt_BW)/1
  Compare To Zero/1 -> Discrete-Time Integrator/2, Discrete-Time Integrator1/2
  Saturation1/1 -> Math Function/1, Product1/2

== system EV_Pwr_Manager/Power_Control/Motor_Limiting/Discharge Power Limit Control/Clamp ==
  preSat : Inport
  saturated : Inport  Port=2
  preIntegrator : Inport  Port=3
  AND : Logic  OutDataTypeStr=boolean
  Compare To Zero : simulink/Logic and Bit Operations/Compare To Zero  relop=<=  OutDataTypeStr=boolean
  Compare To Zero1 : simulink/Logic and Bit Operations/Compare To Zero  relop=<=  OutDataTypeStr=boolean
  Logical Operator : Logic  Operator=NXOR  AllPortsSameDT=off  OutDataTypeStr=boolean
  Clamp : Outport
  wires:
  AND/1 -> Clamp/1
  saturated/1 -> AND/2
  preIntegrator/1 -> Compare To Zero/1
  preSat/1 -> Compare To Zero1/1
  Logical Operator/1 -> AND/1
  Compare To Zero/1 -> Logical Operator/1
  Compare To Zero1/1 -> Logical Operator/2

== system EV_Pwr_Manager/Power_Control/Motor_Limiting/Discharge Power Limit Control/PI_Sat ==
  In1 : Inport
  Dynamic Saturation : Subsystem
      mask Display: plot([0.15 0.85],[.5 .5],[.5 .5],[0.05 0.95],0.15+0.7*[0 .25 .75 1],0.05+0.9*[.25 .25 .75 .75]);
  PI_Sat : Constant  Value=single(EV_Param.Battery_Det.DischargePowerPISat)*1.5  PreserveConstantTs=on
  PI_Sat1 : Constant  Value=single(EV_Param.Battery_Det.DischargePowerPISat)*.25  PreserveConstantTs=on
  Unary Minus : UnaryMinus
  Out1 : Outport
  saturated : Outport  Port=2
  wires:
  Dynamic Saturation/2(sat_mode) -> saturated/1
  Dynamic Saturation/1(y) -> Out1/1
  PI_Sat/1 -> Dynamic Saturation/1(up)
  In1/1 -> Dynamic Saturation/2(u)
  Unary Minus/1 -> Dynamic Saturation/3(lo)
  PI_Sat1/1 -> Unary Minus/1

== system EV_Pwr_Manager/Power_Control/Regen_Limiting/Charge Power Limit Control/Clamp ==
  preSat : Inport
  saturated : Inport  Port=2
  preIntegrator : Inport  Port=3
  AND : Logic  OutDataTypeStr=boolean
  Compare To Zero : simulink/Logic and Bit Operations/Compare To Zero  relop=<=  OutDataTypeStr=boolean
  Compare To Zero1 : simulink/Logic and Bit Operations/Compare To Zero  relop=<=  OutDataTypeStr=boolean
  Logical Operator : Logic  Operator=NXOR  AllPortsSameDT=off  OutDataTypeStr=boolean
  Clamp : Outport
  wires:
  AND/1 -> Clamp/1
  saturated/1 -> AND/2
  preIntegrator/1 -> Compare To Zero/1
  preSat/1 -> Compare To Zero1/1
  Logical Operator/1 -> AND/1
  Compare To Zero/1 -> Logical Operator/1
  Compare To Zero1/1 -> Logical Operator/2

== system EV_Pwr_Manager/Power_Control/Regen_Limiting/Charge Power Limit Control/PI_Sat ==
  In1 : Inport
  Dynamic Saturation : Subsystem
      mask Display: plot([0.15 0.85],[.5 .5],[.5 .5],[0.05 0.95],0.15+0.7*[0 .25 .75 1],0.05+0.9*[.25 .25 .75 .75]);
  PI_Sat : Constant  Value=single(EV_Param.Battery_Det.ChargePowerPISat)  PreserveConstantTs=on
  Unary Minus : UnaryMinus
  Out1 : Outport
  saturated : Outport  Port=2
  wires:
  Dynamic Saturation/2(sat_mode) -> saturated/1
  Dynamic Saturation/1(y) -> Out1/1
  PI_Sat/1 -> Unary Minus/1, Dynamic Saturation/1(up)
  In1/1 -> Dynamic Saturation/2(u)
  Unary Minus/1 -> Dynamic Saturation/3(lo)

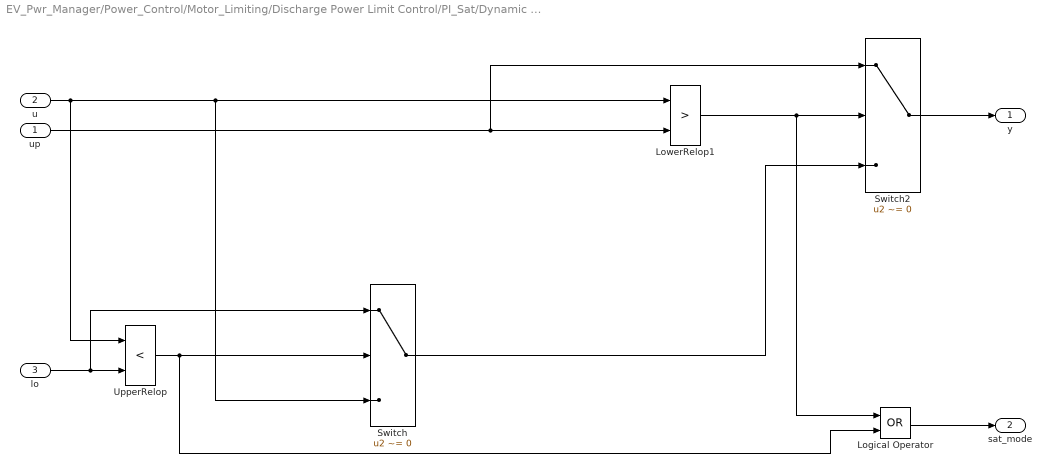
== system EV_Pwr_Manager/Power_Control/Motor_Limiting/Discharge Power Limit Control/PI_Sat/Dynamic Saturation ==
  up : Inport
  u : Inport  Port=2
  lo : Inport  Port=3
  Logical Operator : Logic  Operator=OR  AllPortsSameDT=off  OutDataTypeStr=boolean
  LowerRelop1 : RelationalOperator  DisableCoverage=on  Operator=>  OutDataTypeStr=boolean
  Switch : Switch  Criteria=u2 ~= 0  ZeroCross=off
  Switch2 : Switch  Criteria=u2 ~= 0  ZeroCross=off
  UpperRelop : RelationalOperator  DisableCoverage=on  Operator=<  OutDataTypeStr=boolean
  y : Outport
  sat_mode : Outport  Port=2
  wires:
  Logical Operator/1 -> sat_mode/1
  up/1 -> Switch2/1, LowerRelop1/2
  u/1 -> LowerRelop1/1, Switch/3, UpperRelop/1
  lo/1 -> Switch/1, UpperRelop/2
  Switch/1 -> Switch2/3
  Switch2/1 -> y/1
  LowerRelop1/1 -> Switch2/2, Logical Operator/1
  UpperRelop/1 -> Switch/2, Logical Operator/2

== system EV_Pwr_Manager/Power_Control/Regen_Limiting/Charge Power Limit Control/PI_Sat/Dynamic Saturation ==
  up : Inport
  u : Inport  Port=2
  lo : Inport  Port=3
  Logical Operator : Logic  Operator=OR  AllPortsSameDT=off  OutDataTypeStr=boolean
  LowerRelop1 : RelationalOperator  DisableCoverage=on  Operator=>  OutDataTypeStr=boolean
  Switch : Switch  Criteria=u2 ~= 0  ZeroCross=off
  Switch2 : Switch  Criteria=u2 ~= 0  ZeroCross=off
  UpperRelop : RelationalOperator  DisableCoverage=on  Operator=<  OutDataTypeStr=boolean
  y : Outport
  sat_mode : Outport  Port=2
  wires:
  Logical Operator/1 -> sat_mode/1
  up/1 -> Switch2/1, LowerRelop1/2
  u/1 -> LowerRelop1/1, Switch/3, UpperRelop/1
  lo/1 -> Switch/1, UpperRelop/2
  Switch/1 -> Switch2/3
  Switch2/1 -> y/1
  LowerRelop1/1 -> Switch2/2, Logical Operator/1
  UpperRelop/1 -> Switch/2, Logical Operator/2

== stateflow chart EV_Pwr_Manager/Vehicle Speed Controller/Chart1 ==
  state Stop
    en: Mode=0;
    en: BrakeSet = 1;
  state Accel
    en: Mode=1;
  state Coast
    en: Mode = 2;
  state Decel
    en: Mode = 3;
  (default) -> Stop
  Stop -> (junction 36) : [(Accel_Cmd>0.05)]
      | {BrakeSet=0;}
  (junction 36) -> Accel
  (junction 32) -> Stop
  Decel -> (junction 32) [order 1] : [veh_spd<0.05 && after(200,tick)]
  (junction 34) -> Stop
  Accel -> (junction 34) [order 2] : [veh_spd<0.05...
      |  && Accel_Cmd<0.005]
  Coast -> Stop [order 3] : [veh_spd<0.05 &&...
      | Decel_Cmd<0.05 && ...
      | Accel_Cmd <=0.05 &&...
      |  after(200,tick)]
  Accel -> Coast [order 1] : [Accel_Cmd<0.05 ...
      | && Decel_Cmd <= 1]
  Decel -> Coast [order 2] : [Decel_Cmd<0.5*(veh_spd+1)/40 ...
      | && Accel_Cmd <=1 && veh_spd>1 ]
  Coast -> Decel [order 1] : [(Decel_Cmd>0.75*(veh_spd+1)/10 )]
  Coast -> Accel [order 2] : [(Accel_Cmd>0.125/2)]
  (junction 43) -> Accel
  Accel -> (junction 39) [order 3] : [Accel_Cmd == 0 && Decel_Cmd > 1]
  (junction 40) -> Decel
  Decel -> (junction 38) [order 3] : [Accel_Cmd>1 && Decel_Cmd ==0 && veh_spd>1]
  (junction 39) -> (junction 40)
  (junction 38) -> (junction 43)
  data: Mode output uint8 =0; Accel_Cmd input; Decel_Cmd input; veh_spd input; BrakeSet output boolean
